simulink library "libPilotCmds"  (R2020b)
settings: Solver=VariableStepAuto  StartTime=0.0  StopTime=10.0  RelTol=1e-3
libraries: vrlib x1
settings Model: Creator=caatay  LastModifiedBy=caatay

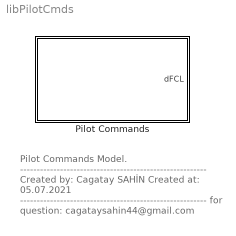
== system libPilotCmds ==
  note: Pilot Commands Model.
      | --------------------------------------------------------
      | Created by: Cagatay SAHİN
      | Created at: 05.07.2021
      | --------------------------------------------------------
      | for question:
      | cagataysahin44@gmail.com
  Pilot Commands : Subsystem  mask(Animation Model - Pilot Commands Model){}
      mask help: Pilot Commands of aircraft that is taken from joystick inputs.
      mask Help:
      | This block is used for get pilot commands from joystick in whole simulation.
      | --------------------------------------------------------------------------------------------------------------------------------------------------
      | --------------------------------------------------------------------------------------------------------------------------------------------------
      | for question: "cagataysahin44@gmail.com"

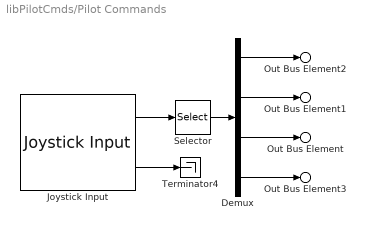
== system libPilotCmds/Pilot Commands ==
  Demux : Demux
  Joystick Input : vrlib/Joystick Input  joyid=1  adjustports=on  forcefeed=off
  Selector : Selector  InputPortWidth=8  IndexOptions=Index vector (dialog)  Indices=[1 2 3 6]  OutputSizes=1
  Terminator4 : Terminator
  Out Bus Element : Outport  PortName=dFCL  Element=throttleCmd
  Out Bus Element1 : Outport  PortName=dFCL  Element=pitch
  Out Bus Element2 : Outport  PortName=dFCL  Element=roll
  Out Bus Element3 : Outport  PortName=dFCL  Element=yaw
  wires:
  Joystick Input/1 -> Selector/1
  Selector/1 -> Demux/1
  Joystick Input/2 -> Terminator4/1
  Demux/3 -> Out Bus Element/1
  Demux/2 -> Out Bus Element1/1
  Demux/1 -> Out Bus Element2/1
  Demux/4 -> Out Bus Element3/1
